simulink model "control"  (R2020a)
settings: Solver=FixedStepDiscrete  StartTime=0.0  StopTime=1  FixedStep=0.0005  RelTol=1e-3  EnableMultiTasking=on
undefined symbols (not defined in the file): acc_calmax1, acc_calmax2, acc_calmin1, acc_calmin2, akemancanshu, bre, bre_calmax, bre_calmin, ecucoder_acal, I_AN01_5K1, I_AN03_5V, I_AN04_5V, kd, ki, kp, leftmax, O_SW06_HS1A, rightmax, T_add, T_del, tiaoshi, zhiling
libraries: ec5744lib x252, canmsglib x92, simulink x5
(part 2 of 9)

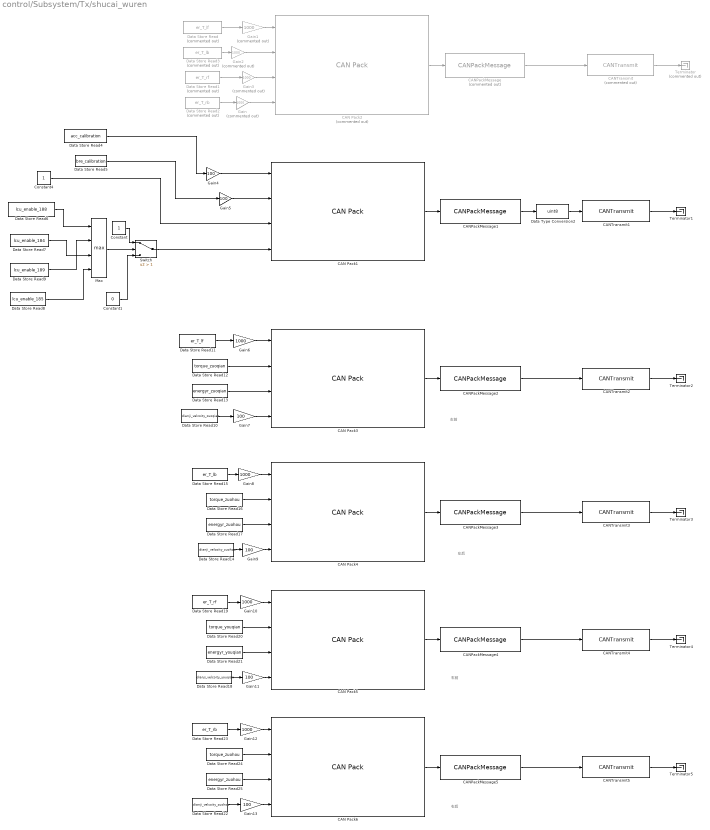
== system control/Subsystem/Tx/shucai_wuren ==
  note: 右后
  note: 右前
  note: 左后
  note: 左前
  CAN Pack1 : canmsglib/CAN Pack  CANdbFile=C:\Users\18137\Desktop\HRT\E02\HRT_23E.dbc  MsgList=(none)  MsgName=shucai  MsgIDType=Standard (11-bit identifier)  MsgIdentifier=5  MsgLength=8  Remote=off  ApplyMinMax=off  BusOutput=off  SignalInfo={'acc_signal','0','8','LE','unsigned','Standard','0','1','0','0','255';'bre_signal','8','8','LE','unsigned','Standard','0','1','0','0','255';'code_version','16','8','LE','unsigned','Standard','0','1','0','0','255';'enable_condition','24','8','LE','unsigned','Standard','0','1','0','0','255'}
      settings: SourceProductBaseCode=ME,XP,VN  DataFormat=CANdb specified signals
  CAN Pack2 : canmsglib/CAN Pack  Commented=on  CANdbFile=C:\Users\18137\Desktop\HRT\E02\HRT_23E.dbc  MsgList=(none)  MsgName=shucai_wuren  MsgIDType=Standard (11-bit identifier)  MsgIdentifier=102  MsgLength=8  Remote=off  ApplyMinMax=off  BusOutput=off  SignalInfo={'current_torque_lf','16','16','LE','signed','Standard','0','1','0','-32768','32767';'current_torque_lr','32','16','LE','signed','Standard','0','1','0','-32768','32767';'current_torque_rf','48','16','LE','signed','Standard','0','1','0','-32768','32767';'current_torque_rr','0','16','LE','signed','Standard','0','1','0','-32768','32767'}
      settings: SourceProductBaseCode=ME,XP,VN  DataFormat=CANdb specified signals
  CAN Pack{3..6} (4 alike) : canmsglib/CAN Pack  CANdbFile=C:\Users\86155\Desktop\HRT2024\qkx\can\energy_receive.dbc  MsgList=caijishuju_Copy_lf  MsgName=caijishuju_Copy_lf  MsgIDType=Standard (11-bit identifier)  MsgIdentifier=257  MsgLength=8  Remote=off  ApplyMinMax=off  BusOutput=off  SignalInfo={'current','0','16','LE','signed','Standard','0','1','0','-32768','32767';'odd_pressure','16','16','LE','signed','Standard','0','1','0','-32768','32767';'torque','32','16','LE','signed','Standard','0','1','0','-32768','32767';'velocity','48','16','LE','signed','Standard','0','1','0','-32768','32767'}
      settings: SourceProductBaseCode=ME,XP,VN  DataFormat=CANdb specified signals
  CANPackMessage : ec5744lib/RapidECU_U4B/04CANCommunication/CANPackMessage  Commented=on  datalength=8  sampletime=-1
      settings: SourceProductName=ECUCoder for MPC5744
  CANPackMessage{1..5} (5 alike) : ec5744lib/RapidECU_U4B/04CANCommunication/CANPackMessage  datalength=8  sampletime=-1
      settings: SourceProductName=ECUCoder for MPC5744
  CANTransmit : ec5744lib/RapidECU_U4B/04CANCommunication/CANTransmit  Commented=on  canmodule=1  canbuffer=8  canmessageid=hex2dec('66')  canmessagetype=Standard(11-bit ID)  datalength=8  sampletime=-1
      settings: SourceProductName=ECUCoder for MPC5744
  CANTransmit1 : ec5744lib/RapidECU_U4B/04CANCommunication/CANTransmit  canmodule=1  canbuffer=57  canmessageid=hex2dec('5')  canmessagetype=Standard(11-bit ID)  datalength=8  sampletime=-1
      settings: SourceProductName=ECUCoder for MPC5744
  CANTransmit2 : ec5744lib/RapidECU_U4B/04CANCommunication/CANTransmit  canmodule=1  canbuffer=58  canmessageid=hex2dec('100')  canmessagetype=Standard(11-bit ID)  datalength=8  sampletime=-1
      settings: SourceProductName=ECUCoder for MPC5744
  CANTransmit3 : ec5744lib/RapidECU_U4B/04CANCommunication/CANTransmit  canmodule=1  canbuffer=59  canmessageid=hex2dec('101')  canmessagetype=Standard(11-bit ID)  datalength=8  sampletime=-1
      settings: SourceProductName=ECUCoder for MPC5744
  CANTransmit4 : ec5744lib/RapidECU_U4B/04CANCommunication/CANTransmit  canmodule=1  canbuffer=60  canmessageid=hex2dec('102')  canmessagetype=Standard(11-bit ID)  datalength=8  sampletime=-1
      settings: SourceProductName=ECUCoder for MPC5744
  CANTransmit5 : ec5744lib/RapidECU_U4B/04CANCommunication/CANTransmit  canmodule=1  canbuffer=61  canmessageid=hex2dec('103')  canmessagetype=Standard(11-bit ID)  datalength=8  sampletime=-1
      settings: SourceProductName=ECUCoder for MPC5744
  Constant : Constant
  Constant1 : Constant  Value=0
  Constant4 : Constant
  Data Store Read : DataStoreRead  Commented=on  DataStoreName=er_T_lf
  Data Store Read1 : DataStoreRead  Commented=on  DataStoreName=er_T_rf
  Data Store Read10 : DataStoreRead  DataStoreName=dianji_velcoity_zuoqian
  Data Store Read11 : DataStoreRead  DataStoreName=er_T_lf
  Data Store Read12 : DataStoreRead  DataStoreName=torque_zuoqian
  Data Store Read13 : DataStoreRead  DataStoreName=energyr_zuoqian
  Data Store Read14 : DataStoreRead  DataStoreName=dianji_velcoity_zuohou
  Data Store Read15 : DataStoreRead  DataStoreName=er_T_lb
  Data Store Read16 : DataStoreRead  DataStoreName=torque_zuohou
  Data Store Read17 : DataStoreRead  DataStoreName=energyr_zuohou
  Data Store Read18 : DataStoreRead  DataStoreName=dianji_velcoity_youqian
  Data Store Read19 : DataStoreRead  DataStoreName=er_T_rf
  Data Store Read2 : DataStoreRead  Commented=on  DataStoreName=er_T_rb
  Data Store Read20 : DataStoreRead  DataStoreName=torque_youqian
  Data Store Read21 : DataStoreRead  DataStoreName=energyr_youqian
  Data Store Read22 : DataStoreRead  DataStoreName=dianji_velcoity_zuohou
  Data Store Read23 : DataStoreRead  DataStoreName=er_T_rb
  Data Store Read24 : DataStoreRead  DataStoreName=torque_zuohou
  Data Store Read25 : DataStoreRead  DataStoreName=energyr_zuohou
  Data Store Read3 : DataStoreRead  Commented=on  DataStoreName=er_T_lb
  Data Store Read4 : DataStoreRead  DataStoreName=acc_calibration
  Data Store Read5 : DataStoreRead  DataStoreName=bre_calibration
  Data Store Read6 : DataStoreRead  DataStoreName=lcu_enable_188
  Data Store Read7 : DataStoreRead  DataStoreName=lcu_enable_184
  Data Store Read8 : DataStoreRead  DataStoreName=lcu_enable_185
  Data Store Read9 : DataStoreRead  DataStoreName=lcu_enable_189
  Data Type Conversion2 : DataTypeConversion  OutDataTypeStr=uint8
  Gain{,1..3} (4 alike) : Gain  Commented=on  Gain=1000
  Gain{6,8,10,12} (4 alike) : Gain  Gain=1000
  Gain{4..5,7,9,11,13} (6 alike) : Gain  Gain=100
  Max : MinMax  Function=max  Inputs=4
  Switch : Switch  Criteria=u2 > Threshold  Threshold=1
  Terminator : Terminator  Commented=on
  Terminator{1..5} (5 alike) : Terminator
  wires:
  CANTransmit/1 -> Terminator/1
  CAN Pack2/1 -> CANPackMessage/1
  CANPackMessage/1 -> CANTransmit/1
  Data Store Read/1 -> Gain1/1
  Data Store Read3/1 -> Gain2/1
  Data Store Read1/1 -> Gain3/1
  Data Store Read2/1 -> Gain/1
  Gain/1 -> CAN Pack2/4
  Gain3/1 -> CAN Pack2/3
  Gain2/1 -> CAN Pack2/2
  Gain1/1 -> CAN Pack2/1
  Gain4/1 -> CAN Pack1/1
  Data Store Read8/1 -> Max/4
  Gain5/1 -> CAN Pack1/2
  CANPackMessage1/1 -> Data Type Conversion2/1
  Data Store Read5/1 -> Gain5/1
  Constant4/1 -> CAN Pack1/3
  Data Store Read9/1 -> Max/2
  Data Store Read6/1 -> Max/1
  Constant1/1 -> Switch/3
  CANTransmit1/1 -> Terminator1/1
  Data Store Read7/1 -> Max/3
  CAN Pack1/1 -> CANPackMessage1/1
  Max/1 -> Switch/2
  Constant/1 -> Switch/1
  Data Store Read4/1 -> Gain4/1
  Data Type Conversion2/1 -> CANTransmit1/1
  Switch/1 -> CAN Pack1/4
  CANPackMessage2/1 -> CANTransmit2/1
  CANTransmit2/1 -> Terminator2/1
  CAN Pack3/1 -> CANPackMessage2/1
  Data Store Read10/1 -> Gain7/1
  Data Store Read11/1 -> Gain6/1
  Data Store Read12/1 -> CAN Pack3/2
  Data Store Read13/1 -> CAN Pack3/3
  Data Store Read17/1 -> CAN Pack4/3
  Data Store Read14/1 -> Gain9/1
  Data Store Read15/1 -> Gain8/1
  Data Store Read16/1 -> CAN Pack4/2
  CAN Pack4/1 -> CANPackMessage3/1
  CANTransmit3/1 -> Terminator3/1
  CANPackMessage3/1 -> CANTransmit3/1
  Data Store Read21/1 -> CAN Pack5/3
  Data Store Read18/1 -> Gain11/1
  Data Store Read19/1 -> Gain10/1
  Data Store Read20/1 -> CAN Pack5/2
  CAN Pack5/1 -> CANPackMessage4/1
  CANTransmit4/1 -> Terminator4/1
  CANPackMessage4/1 -> CANTransmit4/1
  Data Store Read25/1 -> CAN Pack6/3
  Data Store Read22/1 -> Gain13/1
  Data Store Read23/1 -> Gain12/1
  Data Store Read24/1 -> CAN Pack6/2
  CAN Pack6/1 -> CANPackMessage5/1
  CANTransmit5/1 -> Terminator5/1
  CANPackMessage5/1 -> CANTransmit5/1
  Gain6/1 -> CAN Pack3/1
  Gain7/1 -> CAN Pack3/4
  Gain8/1 -> CAN Pack4/1
  Gain9/1 -> CAN Pack4/4
  Gain10/1 -> CAN Pack5/1
  Gain11/1 -> CAN Pack5/4
  Gain12/1 -> CAN Pack6/1
  Gain13/1 -> CAN Pack6/4

== system control/Subsystem/Tx/转向 ==
  Data Store Read1 : DataStoreRead  DataStoreName=match_model
  Data Store Read2 : DataStoreRead  DataStoreName=status
  Data Store Write : DataStoreWrite  DataStoreName=kp
  Data Store Write1 : DataStoreWrite  DataStoreName=ki
  Data Store Write2 : DataStoreWrite  DataStoreName=kd
  Data Store Write3 : DataStoreWrite  DataStoreName=kenable
  ECCalVar : Constant  InitFcn=ecucoder_acal;  Value=kp  OutDataTypeStr=Inherit: Inherit via back propagation  SampleTime=-1
  ECCalVar1 : Constant  InitFcn=ecucoder_acal;  Value=ki  OutDataTypeStr=Inherit: Inherit via back propagation  SampleTime=-1
  ECCalVar2 : Constant  InitFcn=ecucoder_acal;  Value=kd  OutDataTypeStr=Inherit: Inherit via back propagation  SampleTime=-1
  MATLAB Function1 : MATLAB Function  TreatAsAtomicUnit=on
  Max : MinMax  Inputs=3
  转向换算 : Subsystem
  wires:
  Data Store Read1/1 -> MATLAB Function1/1(model)
  ECCalVar1/1 -> Max/2, Data Store Write1/1
  ECCalVar2/1 -> Max/1, Data Store Write2/1
  ECCalVar/1 -> Max/3, Data Store Write/1
  Data Store Read2/1 -> MATLAB Function1/2(status)
  MATLAB Function1/1(y) -> 转向换算/Enable
  Max/1 -> Data Store Write3/1

== system control/Subsystem/run/analog_input ==
  Add : Sum
  Data Store Read{,1..3,7} (5 alike) : DataStoreRead  DataStoreName=match_model
  Data Store Read4 : DataStoreRead  DataStoreName=lcu_canok
  Data Store Read5 : DataStoreRead  DataStoreName=lcu_canok
  Data Store Read6 : DataStoreRead  DataStoreName=workstation_status
  Data Store Read8 : DataStoreRead  DataStoreName=V_workstation
  Data Store Read9 : DataStoreRead  DataStoreName=V_Kalman
  MATLAB Function : MATLAB Function  TreatAsAtomicUnit=on
  MATLAB Function1 : MATLAB Function  TreatAsAtomicUnit=on
  MATLAB Function2 : MATLAB Function  TreatAsAtomicUnit=on
  MATLAB Function3 : MATLAB Function  TreatAsAtomicUnit=on
  MATLAB Function4 : MATLAB Function  TreatAsAtomicUnit=on
  MATLAB Function5 : MATLAB Function  TreatAsAtomicUnit=on
  MATLAB Function6 : MATLAB Function  TreatAsAtomicUnit=on
  Saturation : Saturate  UpperLimit=50  LowerLimit=0
  Switch : Switch  Criteria=u2 > Threshold
  基准扭矩 : DataStoreWrite  Commented=on  DataStoreName=M
  无人意图转译 : Subsystem
  有人 : Subsystem
  bre : Outport
  acc : Outport  Port=2
  wires:
  Data Store Read1/1 -> MATLAB Function/1(u)
  MATLAB Function/1(y) -> MATLAB Function1/1(u)
  Switch/1 -> MATLAB Function1/2(a)
  有人/1(TP) -> Switch/3
  有人/2(bre) -> bre/1
  Data Store Read2/1 -> MATLAB Function2/1(u)
  MATLAB Function2/1(y) -> 有人/Enable
  Data Store Read3/1 -> MATLAB Function3/1(model)
  无人意图转译/1(Out1) -> Switch/1
  MATLAB Function3/1(y) -> 无人意图转译/Enable
  Data Store Read4/1 -> MATLAB Function3/2(canok)
  Data Store Read5/1 -> MATLAB Function2/2(canok)
  Data Store Read6/1 -> MATLAB Function4/1(u)
  MATLAB Function1/1(y) -> MATLAB Function4/2(a)
  MATLAB Function4/1(y) -> MATLAB Function5/1(u)
  Data Store Read7/1 -> MATLAB Function5/2(model)
  MATLAB Function5/2(y6) -> Saturation/1
  Saturation/1 -> Add/2
  MATLAB Function5/1(y) -> Add/1
  Add/1 -> 基准扭矩/1, acc/1
  MATLAB Function6/1(y) -> Switch/2
  Data Store Read8/1 -> MATLAB Function3/3(workstation)
  Data Store Read9/1 -> MATLAB Function3/4(v)
  Data Store Read/1 -> MATLAB Function6/1(model)

== system control/Subsystem/run/ctrl ==
  note: 控制策略所在地
  基准扭矩 : Inport
  Subsystem1 : Subsystem
  wires:
  基准扭矩/1 -> Subsystem1/1(扭矩)

== system control/无人TX1/转向自动标定/Subsystem ==
  Enable : EnablePort
  CAN Pack : canmsglib/CAN Pack  CANdbFile=C:\Users\Liu keliang\Desktop\HRT2023\HRT23赛季刘科良\CANdbc\steering.dbc  MsgList=(none)  MsgName=enable123  MsgIDType=Standard (11-bit identifier)  MsgIdentifier=291  MsgLength=1  Remote=off  ApplyMinMax=off  BusOutput=off  SignalInfo={'enable123','0','8','LE','unsigned','Standard','0','1','0','0','255'}
      settings: SourceProductBaseCode=ME,XP,VN  DataFormat=CANdb specified signals
  CAN Pack1 : canmsglib/CAN Pack  CANdbFile=C:\Users\Liu keliang\Desktop\HRT2023\HRT23赛季刘科良\CANdbc\steering.dbc  MsgList=(none)  MsgName=enable0  MsgIDType=Standard (11-bit identifier)  MsgIdentifier=0  MsgLength=8  Remote=off  ApplyMinMax=off  BusOutput=off  SignalInfo={'enable_00','0','16','LE','unsigned','Standard','0','1','0','0','65535';'enable_00_Copy_1','16','16','LE','unsigned','Standard','0','1','0','0','65535';'enable_00_Copy_2','32','16','LE','unsigned','Standard','0','1','0','0','65535';'enable_00_Copy_3','48','16','LE','unsigned','Standard','0','1','0','0','65535'}
      settings: SourceProductBaseCode=ME,XP,VN  DataFormat=CANdb specified signals
  CAN Pack2 : canmsglib/CAN Pack  CANdbFile=C:\Users\Liu keliang\Desktop\HRT2023\HRT23赛季刘科良\CANdbc\steering.dbc  MsgList=(none)  MsgName=enable401  MsgIDType=Standard (11-bit identifier)  MsgIdentifier=1025  MsgLength=6  Remote=off  ApplyMinMax=off  BusOutput=off  SignalInfo={'enable401','0','8','LE','unsigned','Standard','0','1','0','0','255';'enable401_Copy_1','8','8','LE','unsigned','Standard','0','1','0','0','255';'enable401_Copy_2','16','32','LE','signed','Standard','0','1','0','-2147483648','2147483647'}
      settings: SourceProductBaseCode=ME,XP,VN  DataFormat=CANdb specified signals
  CAN Pack4 : canmsglib/CAN Pack  CANdbFile=C:\Users\Liu keliang\Desktop\HRT2023\HRT23赛季刘科良\CANdbc\steering.dbc  MsgList=(none)  MsgName=enable80  MsgIDType=Standard (11-bit identifier)  MsgIdentifier=128  MsgLength=1  Remote=off  ApplyMinMax=off  BusOutput=off  SignalInfo={'dingshi','0','8','LE','unsigned','Standard','0','1','0','0','255'}
      settings: SourceProductBaseCode=ME,XP,VN  DataFormat=CANdb specified signals
  CANPackMessage : ec5744lib/RapidECU_U4B/04CANCommunication/CANPackMessage  datalength=1  sampletime=-1
      settings: SourceProductName=ECUCoder for MPC5744
  CANPackMessage1 : ec5744lib/RapidECU_U4B/04CANCommunication/CANPackMessage  datalength=8  sampletime=-1
      settings: SourceProductName=ECUCoder for MPC5744
  CANPackMessage2 : ec5744lib/RapidECU_U4B/04CANCommunication/CANPackMessage  datalength=6  sampletime=-1
      settings: SourceProductName=ECUCoder for MPC5744
  CANPackMessage4 : ec5744lib/RapidECU_U4B/04CANCommunication/CANPackMessage  datalength=1  sampletime=-1
      settings: SourceProductName=ECUCoder for MPC5744
  CANTransmit : ec5744lib/RapidECU_U4B/04CANCommunication/CANTransmit  canmodule=2  canbuffer=15  canmessageid=hex2dec('123')  canmessagetype=Standard(11-bit ID)  datalength=1  sampletime=-1
      settings: SourceProductName=ECUCoder for MPC5744
  CANTransmit1 : ec5744lib/RapidECU_U4B/04CANCommunication/CANTransmit  canmodule=2  canbuffer=56  canmessageid=hex2dec('00')  canmessagetype=Standard(11-bit ID)  datalength=8  sampletime=-1
      settings: SourceProductName=ECUCoder for MPC5744
  CANTransmit2 : ec5744lib/RapidECU_U4B/04CANCommunication/CANTransmit  canmodule=2  canbuffer=57  canmessageid=hex2dec('401')  canmessagetype=Standard(11-bit ID)  datalength=6  sampletime=-1
      settings: SourceProductName=ECUCoder for MPC5744
  CANTransmit4 : ec5744lib/RapidECU_U4B/04CANCommunication/CANTransmit  canmodule=2  canbuffer=58  canmessageid=hex2dec('80')  canmessagetype=Standard(11-bit ID)  datalength=1  sampletime=-1
      settings: SourceProductName=ECUCoder for MPC5744
  Constant : Constant  Value=0  SampleTime=-1
  Constant1 : Constant  SampleTime=-1
  Constant{2..4,6} (4 alike) : Constant  Value=0
  Constant5 : Constant  Value=0  SampleTime=-1
  Data Store Read : DataStoreRead  DataStoreName=zhuanjiaobianmaqi
  Data Store Read1 : DataStoreRead  DataStoreName=rm
  Data Store Read2 : DataStoreRead  DataStoreName=lm
  Data Type Conversion : DataTypeConversion  OutDataTypeStr=uint8
  Data Type Conversion1 : DataTypeConversion  OutDataTypeStr=uint8
  Data Type Conversion2 : DataTypeConversion  Commented=on  OutDataTypeStr=uint8
  Data Type Conversion3 : DataTypeConversion  OutDataTypeStr=single
  Data Type Conversion4 : DataTypeConversion  OutDataTypeStr=uint8
  Data Type Conversion5 : DataTypeConversion  OutDataTypeStr=single
  Data Type Conversion6 : DataTypeConversion  OutDataTypeStr=single
  FRAMEnable : ec5744lib/RapidECU_U4B/12EEModule/FRAMEnable  framenable=on
      settings: SourceProductName=ECUCoder for MPC5744
  FRAMWrite : ec5744lib/RapidECU_U4B/12EEModule/FRAMWrite  buffer=0  sampletime=-1
      settings: SourceProductName=ECUCoder for MPC5744
  FRAMWrite1 : ec5744lib/RapidECU_U4B/12EEModule/FRAMWrite  buffer=1  sampletime=-1
      settings: SourceProductName=ECUCoder for MPC5744
  FRAMWrite2 : ec5744lib/RapidECU_U4B/12EEModule/FRAMWrite  buffer=10  sampletime=-1
      settings: SourceProductName=ECUCoder for MPC5744
  FRAMWrite3 : ec5744lib/RapidECU_U4B/12EEModule/FRAMWrite  buffer=11  sampletime=-1
      settings: SourceProductName=ECUCoder for MPC5744
  MATLAB Function : MATLAB Function  TreatAsAtomicUnit=on
  MeaModule : ec5744lib/RapidECU_U4B/07Calibration/MeaModule  signal=msk
      settings: SourceProductName=ECUCoder for MPC5744
  MeaModule1 : ec5744lib/RapidECU_U4B/07Calibration/MeaModule  signal=msd
      settings: SourceProductName=ECUCoder for MPC5744
  Terminator{,1..2,4} (4 alike) : Terminator
  Zero-Order Hold{,1..4} (5 alike) : ZeroOrderHold  SampleTime=-1
  wires:
  CANTransmit/1 -> Terminator/1
  Zero-Order Hold2/1 -> CAN Pack1/3
  MATLAB Function/2(y) -> CAN Pack2/1
  CAN Pack1/1 -> CANPackMessage1/1
  CANTransmit2/1 -> Terminator2/1
  CANPackMessage4/1 -> Data Type Conversion4/1
  CAN Pack2/1 -> CANPackMessage2/1
  CANTransmit1/1 -> Terminator1/1
  Constant/1 -> Zero-Order Hold/1
  Data Type Conversion1/1 -> CANTransmit1/1
  Constant6/1 -> CAN Pack2/2
  CANTransmit4/1 -> Terminator4/1
  Data Type Conversion/1 -> CANTransmit/1
  Zero-Order Hold/1 -> CAN Pack/1
  CANPackMessage/1 -> Data Type Conversion/1
  Data Type Conversion4/1 -> CANTransmit4/1
  Constant4/1 -> Zero-Order Hold3/1
  CAN Pack/1 -> CANPackMessage/1
  CANPackMessage1/1 -> Data Type Conversion1/1
  Constant5/1 -> Zero-Order Hold4/1
  CAN Pack4/1 -> CANPackMessage4/1
  Constant3/1 -> Zero-Order Hold2/1
  Constant2/1 -> Zero-Order Hold1/1
  Constant1/1 -> CAN Pack1/1
  Zero-Order Hold4/1 -> CAN Pack4/1
  Zero-Order Hold1/1 -> CAN Pack1/2
  CANPackMessage2/1 -> CANTransmit2/1
  Zero-Order Hold3/1 -> CAN Pack1/4
  MATLAB Function/1(steer) -> CAN Pack2/3
  Data Store Read/1 -> Data Type Conversion3/1
  MATLAB Function/3(k) -> MeaModule/1
  Data Store Read1/1 -> FRAMWrite2/1, MATLAB Function/1(rm)
  Data Store Read2/1 -> FRAMWrite3/1, MATLAB Function/2(lm)
  Data Type Conversion3/1 -> MATLAB Function/3(bianmaqi)
  MATLAB Function/4(d) -> MeaModule1/1
  MeaModule1/1 -> Data Type Conversion5/1
  Data Type Conversion5/1 -> FRAMWrite1/1
  Data Type Conversion6/1 -> FRAMWrite/1
  MeaModule/1 -> Data Type Conversion6/1

== system control/无人TX1/转向自动标定/Subsystem1 ==
  y1 : Inport
  y2 : Inport  Port=2
  Enable : EnablePort
  CAN Pack5 : canmsglib/CAN Pack  CANdbFile=C:\Users\Liu keliang\Desktop\HRT2023\HRT23赛季刘科良\CANdbc\zhuanxiangresetting.dbc  MsgList=(none)  MsgName=reseting  MsgIDType=Standard (11-bit identifier)  MsgIdentifier=1537  MsgLength=8  Remote=off  ApplyMinMax=off  BusOutput=off  SignalInfo={'reseting1','0','32','LE','unsigned','Standard','0','1','0','-Inf','Inf';'reseting2','32','32','LE','unsigned','Standard','0','1','0','-Inf','Inf'}
      settings: SourceProductBaseCode=ME,XP,VN  DataFormat=CANdb specified signals
  CANPackMessage3 : ec5744lib/RapidECU_U4B/04CANCommunication/CANPackMessage  datalength=8  sampletime=-1
      settings: SourceProductName=ECUCoder for MPC5744
  CANTransmit3 : ec5744lib/RapidECU_U4B/04CANCommunication/CANTransmit  canmodule=2  canbuffer=60  canmessageid=hex2dec('601')  canmessagetype=Standard(11-bit ID)  datalength=8  sampletime=-1
      settings: SourceProductName=ECUCoder for MPC5744
  Data Type Conversion3 : DataTypeConversion  OutDataTypeStr=uint8
  Terminator3 : Terminator
  wires:
  CAN Pack5/1 -> CANPackMessage3/1
  y1/1 -> CAN Pack5/1
  CANTransmit3/1 -> Terminator3/1
  Data Type Conversion3/1 -> CANTransmit3/1
  CANPackMessage3/1 -> Data Type Conversion3/1
  y2/1 -> CAN Pack5/2

== system control/Subsystem/Rx/283 285左前/Subsystem1 ==
  Enable : Inport
  ID : Inport  Port=2
  msg : Inport  Port=3
  function : TriggerPort  TriggerType=function-call  VariantControl=Variant
  Subsystem : Subsystem
  wires:
  ID/1 -> Subsystem/1(ID)
  msg/1 -> Subsystem/2(msg)
  Enable/1 -> Subsystem/Enable

== system control/Subsystem/Rx/283 285左前/Subsystem2 ==
  Enable : Inport
  ID : Inport  Port=2
  msg : Inport  Port=3
  function : TriggerPort  TriggerType=function-call  VariantControl=Variant
  Subsystem : Subsystem
  wires:
  ID/1 -> Subsystem/1(ID)
  msg/1 -> Subsystem/2(msg)
  Enable/1 -> Subsystem/Enable

== system control/Subsystem/Rx/284 286右前/Subsystem1 ==
  Enable : Inport
  ID : Inport  Port=2
  msg : Inport  Port=3
  function : TriggerPort  TriggerType=function-call  VariantControl=Variant
  Subsystem : Subsystem
  wires:
  ID/1 -> Subsystem/1(ID)
  msg/1 -> Subsystem/2(msg)
  Enable/1 -> Subsystem/Enable

== system control/Subsystem/Rx/284 286右前/Subsystem2 ==
  Enable : Inport
  ID : Inport  Port=2
  msg : Inport  Port=3
  function : TriggerPort  TriggerType=function-call  VariantControl=Variant
  Subsystem : Subsystem
  wires:
  ID/1 -> Subsystem/1(ID)
  msg/1 -> Subsystem/2(msg)
  Enable/1 -> Subsystem/Enable

== system control/Subsystem/Rx/287 289右后/Subsystem1 ==
  Enable : Inport
  ID : Inport  Port=2
  msg : Inport  Port=3
  function : TriggerPort  TriggerType=function-call  VariantControl=Variant
  Subsystem : Subsystem
  wires:
  ID/1 -> Subsystem/1(ID)
  msg/1 -> Subsystem/2(msg)
  Enable/1 -> Subsystem/Enable

== system control/Subsystem/Rx/287 289右后/Subsystem3 ==
  Enable : Inport
  ID : Inport  Port=2
  msg : Inport  Port=3
  function : TriggerPort  TriggerType=function-call  VariantControl=Variant
  Subsystem : Subsystem
  wires:
  ID/1 -> Subsystem/1(ID)
  msg/1 -> Subsystem/2(msg)
  Enable/1 -> Subsystem/Enable

== system control/Subsystem/Rx/288 290左后/Subsystem1 ==
  Enable : Inport
  ID : Inport  Port=2
  msg : Inport  Port=3
  function : TriggerPort  TriggerType=function-call  VariantControl=Variant
  Subsystem : Subsystem
  wires:
  ID/1 -> Subsystem/1(ID)
  msg/1 -> Subsystem/2(msg)
  Enable/1 -> Subsystem/Enable

== system control/Subsystem/Rx/288 290左后/Subsystem2 ==
  Enable : Inport
  ID : Inport  Port=2
  msg : Inport  Port=3
  function : TriggerPort  TriggerType=function-call  VariantControl=Variant
  Subsystem : Subsystem
  wires:
  ID/1 -> Subsystem/1(ID)
  msg/1 -> Subsystem/2(msg)
  Enable/1 -> Subsystem/Enable

== system control/Subsystem/Rx/ebs/Subsystem3 ==
  Enable : Inport
  ID : Inport  Port=2
  msg : Inport  Port=3
  function : TriggerPort  TriggerType=function-call  VariantControl=Variant
  Subsystem : Subsystem
  wires:
  ID/1 -> Subsystem/1(ID)
  msg/1 -> Subsystem/2(msg)
  Enable/1 -> Subsystem/Enable

== system control/Subsystem/Rx/lcu——receive/Subsystem1 ==
  Enable : Inport
  ID : Inport  Port=2
  msg : Inport  Port=3
  function : TriggerPort  TriggerType=function-call  VariantControl=Variant
  Subsystem : Subsystem
  m : Outport
  wires:
  ID/1 -> Subsystem/1(ID)
  msg/1 -> Subsystem/2(msg)
  Enable/1 -> Subsystem/Enable
  Subsystem/1(CAN_msg_enable) -> m/1

== system control/Subsystem/Rx/工作站/Subsystem1 ==
  Enable : Inport
  ID : Inport  Port=2
  msg : Inport  Port=3
  function : TriggerPort  TriggerType=function-call  VariantControl=Variant
  Subsystem1 : Subsystem
  wires:
  Enable/1 -> Subsystem1/Enable
  ID/1 -> Subsystem1/1(ID)
  msg/1 -> Subsystem1/2(msg)

== system control/Subsystem/Rx/工作站/Subsystem3 ==
  Enable : Inport
  ID : Inport  Port=2
  msg : Inport  Port=3
  function : TriggerPort  TriggerType=function-call  VariantControl=Variant
  Subsystem : Subsystem
  wires:
  ID/1 -> Subsystem/1(ID)
  msg/1 -> Subsystem/2(msg)
  Enable/1 -> Subsystem/Enable

== system control/Subsystem/Rx/惯导/Subsystem1 ==
  Enable : Inport
  ID : Inport  Port=2
  msg : Inport  Port=3
  function : TriggerPort  TriggerType=function-call  VariantControl=Variant
  Subsystem : Subsystem
  wires:
  ID/1 -> Subsystem/1(ID)
  msg/1 -> Subsystem/2(msg)
  Enable/1 -> Subsystem/Enable

== system control/Subsystem/Rx/惯导/Subsystem2 ==
  Enable : Inport
  ID : Inport  Port=2
  msg : Inport  Port=3
  function : TriggerPort  TriggerType=function-call  VariantControl=Variant
  Subsystem : Subsystem
  wires:
  ID/1 -> Subsystem/1(ID)
  msg/1 -> Subsystem/2(msg)
  Enable/1 -> Subsystem/Enable

== system control/Subsystem/Rx/惯导/Subsystem3 ==
  Enable : Inport
  ID : Inport  Port=2
  msg : Inport  Port=3
  function : TriggerPort  TriggerType=function-call  VariantControl=Variant
  Subsystem : Subsystem
  wires:
  ID/1 -> Subsystem/1(ID)
  msg/1 -> Subsystem/2(msg)
  Enable/1 -> Subsystem/Enable

== system control/Subsystem/Rx/转向——receive1/Subsystem1 ==
  Enable : Inport
  ID : Inport  Port=2
  msg : Inport  Port=3
  function : TriggerPort  TriggerType=function-call  VariantControl=Variant
  Subsystem : Subsystem
  wires:
  ID/1 -> Subsystem/1(ID)
  msg/1 -> Subsystem/2(msg)
  Enable/1 -> Subsystem/Enable

== system control/Subsystem/Rx/转向——receive1/Subsystem3 ==
  Enable : Inport
  ID : Inport  Port=2
  msg : Inport  Port=3
  function : TriggerPort  TriggerType=function-call  VariantControl=Variant
  Subsystem : Subsystem
  wires:
  ID/1 -> Subsystem/1(ID)
  msg/1 -> Subsystem/2(msg)
  Enable/1 -> Subsystem/Enable

== system control/Subsystem/Rx/转向——receive编码器/Subsystem3 ==
  Enable : Inport
  ID : Inport  Port=2
  msg : Inport  Port=3
  function : TriggerPort  TriggerType=function-call  VariantControl=Variant
  Subsystem : Subsystem
  wires:
  ID/1 -> Subsystem/1(ID)
  msg/1 -> Subsystem/2(msg)
  Enable/1 -> Subsystem/Enable

== system control/Subsystem/Tx/TX控制器/Subsystem1 ==
  angle : Inport
  v : Inport  Port=2
  Data Store Read4 : DataStoreRead  DataStoreName=match_model
  ECCalVar : Constant  InitFcn=ecucoder_acal;  Value=akemancanshu  OutDataTypeStr=Inherit: Inherit via back propagation  SampleTime=-1
  MATLAB Function2 : MATLAB Function  TreatAsAtomicUnit=on
  youqianvvv : Outport
  zuoqianvvv : Outport  Port=2
  youhouvvv : Outport  Port=3
  zuohouvvv : Outport  Port=4
  wires:
  MATLAB Function2/2(zuoqianvvv) -> zuoqianvvv/1
  v/1 -> MATLAB Function2/2(v)
  MATLAB Function2/1(youqianvvv) -> youqianvvv/1
  MATLAB Function2/3(youhouvvv) -> youhouvvv/1
  angle/1 -> MATLAB Function2/1(anglenb)
  MATLAB Function2/4(zuohouvvv) -> zuohouvvv/1
  Data Store Read4/1 -> MATLAB Function2/3(model)
  ECCalVar/1 -> MATLAB Function2/4(k)

== system control/Subsystem/Tx/TX控制器/扭矩 ==
  note: 185右前 284 286
  note: 188右后 287 289
  note: 184左前 283 285
  note: 189左后 288 290
  Enable : EnablePort
  184左前 : Subsystem
  185右前 : Subsystem
  188右后 : Subsystem
  189左后 : Subsystem
  TEST : Subsystem  Commented=on

== system control/Subsystem/Tx/TX控制器/速度 ==
  note: 185右前 284 286
  note: 188右后 287 289
  note: 184左前 283 285
  note: 189左后 288 290
  Enable : EnablePort
  184左前 : Subsystem
  185右前 : Subsystem
  188右后 : Subsystem
  189左后 : Subsystem

== system control/Subsystem/Tx/TX控制器/速度1 ==
  note: 189左后 288 290
  note: 184左前 283 285
  note: 188右后 287 289
  note: 185右前 284 286
  Enable : EnablePort
  184左前 : Subsystem
  185右前 : Subsystem
  188右后 : Subsystem
  189左后 : Subsystem

== system control/Subsystem/Tx/Toworkstation/toworkstation ==
  Enable : EnablePort
  toworkstation : Subsystem

== system control/Subsystem/Tx/Toworkstation/转向 ==
  Data Store Read : DataStoreRead  DataStoreName=match_model
  MATLAB Function : MATLAB Function  TreatAsAtomicUnit=on
  Subsystem : Subsystem
  wires:
  Data Store Read/1 -> MATLAB Function/1(u)
  MATLAB Function/1(y) -> Subsystem/Enable

== system control/Subsystem/Tx/esc，ABS/Subsystem ==
  Enable : EnablePort
  CAN Pack : canmsglib/CAN Pack  CANdbFile=C:\Users\Liu keliang\Desktop\HRT2023\HRT23赛季刘科良\CANdbc\esc.dbc  MsgList=(none)  MsgName=esc  MsgIDType=Standard (11-bit identifier)  MsgIdentifier=1638  MsgLength=8  Remote=off  ApplyMinMax=off  BusOutput=off  SignalInfo={'youhou','0','16','LE','unsigned','Standard','0','1','0','0','65535';'youqian','16','16','LE','unsigned','Standard','0','1','0','0','65535';'zuohou','32','16','LE','unsigned','Standard','0','1','0','0','65535';'zuoqian','48','16','LE','unsigned','Standard','0','1','0','0','65535'}
      settings: SourceProductBaseCode=ME,XP,VN  DataFormat=CANdb specified signals
  CANPackMessage : ec5744lib/RapidECU_U4B/04CANCommunication/CANPackMessage  datalength=8  sampletime=-1
      settings: SourceProductName=ECUCoder for MPC5744
  CANTransmit : ec5744lib/RapidECU_U4B/04CANCommunication/CANTransmit  canmodule=2  canbuffer=12  canmessageid=hex2dec('666')  canmessagetype=Standard(11-bit ID)  datalength=8  sampletime=-1
      settings: SourceProductName=ECUCoder for MPC5744
  Data Store Read : DataStoreRead  DataStoreName=oral_pressure_leftbehind
  Data Store Read1 : DataStoreRead  DataStoreName=oral_pressure_rightbehind
  Data Store Read2 : DataStoreRead  DataStoreName=oral_pressure_rightfront
  Data Store Read3 : DataStoreRead  DataStoreName=oral_pressure_leftfront
  Data Store Read4 : DataStoreRead  DataStoreName=brake_slipzuohou
  Data Store Read5 : DataStoreRead  DataStoreName=brake_slipyouhou
  Data Store Read6 : DataStoreRead  DataStoreName=brake_slipyouqian
  Data Store Read7 : DataStoreRead  DataStoreName=brake_slipzuoqian
  Data Store Read8 : DataStoreRead  DataStoreName=workstation_status
  Data Type Conversion : DataTypeConversion  OutDataTypeStr=uint8
  MATLAB Function : MATLAB Function  TreatAsAtomicUnit=on
  MATLAB Function1 : MATLAB Function  TreatAsAtomicUnit=on
  MATLAB Function2 : MATLAB Function  TreatAsAtomicUnit=on
  MATLAB Function3 : MATLAB Function  TreatAsAtomicUnit=on
  Max{,1..3} (4 alike) : MinMax  Function=max  Inputs=2
  MeaModule : ec5744lib/RapidECU_U4B/07Calibration/MeaModule  signal=esc
      settings: SourceProductName=ECUCoder for MPC5744
  Terminator : Terminator
  wires:
  CAN Pack/1 -> CANPackMessage/1
  CANTransmit/1 -> MeaModule/1
  Data Type Conversion/1 -> CANTransmit/1
  CANPackMessage/1 -> Data Type Conversion/1
  MeaModule/1 -> Terminator/1
  Data Store Read5/1 -> Max/1
  Data Store Read1/1 -> Max/2
  Data Store Read2/1 -> Max1/1
  Data Store Read6/1 -> Max1/2
  Data Store Read/1 -> Max2/1
  Data Store Read4/1 -> Max2/2
  Data Store Read7/1 -> Max3/1
  Data Store Read3/1 -> Max3/2
  Data Store Read8/1 -> MATLAB Function/2(status), MATLAB Function1/2(status), MATLAB Function2/2(status), MATLAB Function3/2(status)
  Max1/1 -> MATLAB Function1/1(u)
  Max2/1 -> MATLAB Function2/1(u)
  Max3/1 -> MATLAB Function3/1(u)
  MATLAB Function/1(y) -> CAN Pack/1
  MATLAB Function1/1(y) -> CAN Pack/2
  MATLAB Function2/1(y) -> CAN Pack/3
  MATLAB Function3/1(y) -> CAN Pack/4
  Max/1 -> MATLAB Function/1(u)

== system control/Subsystem/Tx/转向/转向换算 ==
  Enable : EnablePort
  Data Store Read : DataStoreRead  DataStoreName=zhuanxiangbaocuo
  Data Store Read1 : DataStoreRead  DataStoreName=zhuanxiangbaocuo
  MATLAB Function : MATLAB Function  TreatAsAtomicUnit=on
  MATLAB Function1 : MATLAB Function  TreatAsAtomicUnit=on
  Subsystem : Subsystem
  Subsystem1 : Subsystem
  wires:
  MATLAB Function/1(biaozhi1) -> Subsystem/Enable
  MATLAB Function1/3(biaozhi2) -> Subsystem1/Enable
  MATLAB Function1/2(y2) -> Subsystem1/2(y2)
  MATLAB Function1/1(y1) -> Subsystem1/1(y1)
  Data Store Read/1 -> MATLAB Function1/1(baocuo)
  Data Store Read1/1 -> MATLAB Function/1(baocuo)

== system control/Subsystem/run/analog_input/无人意图转译 ==
  note: 输出基准转矩
  Enable : EnablePort
  Data Store Read : DataStoreRead  DataStoreName=CANOK_20
  Saturation : Saturate  UpperLimit=1300  LowerLimit=0
  无人 : Subsystem
  计算期望扭矩 : MATLAB Function  TreatAsAtomicUnit=on
  Out1 : Outport
  wires:
  无人/1(期望纵向加速度) -> 计算期望扭矩/1(u)
  计算期望扭矩/1(y) -> Saturation/1
  Saturation/1 -> Out1/1
  Data Store Read/1 -> 计算期望扭矩/2(canok)

== system control/Subsystem/run/analog_input/有人 ==
  note: 加速踏板信号转化为0-1范围
      | 即开度
  Enable : EnablePort
  Data Store Write : DataStoreWrite  DataStoreName=yourenniuju
  MeaModule9 : ec5744lib/RapidECU_U4B/07Calibration/MeaModule  signal=tttttttt
      settings: SourceProductName=ECUCoder for MPC5744
  Subsystem : Subsystem
  Subsystem1 : Subsystem
  TP : Outport
  bre : Outport  Port=2
  wires:
  Subsystem/2(bre) -> bre/1
  Subsystem/1(acc) -> Subsystem1/1(acc_signal)
  Subsystem1/1(TP) -> MeaModule9/1
  MeaModule9/1 -> Data Store Write/1, TP/1

== system control/Subsystem/run/ctrl/Subsystem1 ==
  扭矩 : Inport
  Data Store Write : DataStoreWrite  DataStoreName=Tzuoqian
  Data Store Write1 : DataStoreWrite  DataStoreName=Tyouhou
  Data Store Write2 : DataStoreWrite  DataStoreName=Tzuohou
  Data Store Write3 : DataStoreWrite  DataStoreName=Tyouqian
  control_strategy : Subsystem
  wires:
  control_strategy/3(zuohou) -> Data Store Write2/1
  扭矩/1 -> control_strategy/1(TP)
  control_strategy/2(youqian) -> Data Store Write3/1
  control_strategy/1(youhou) -> Data Store Write1/1
  control_strategy/4(zuoqian) -> Data Store Write/1

== system control/Subsystem/Rx/283 285左前/Subsystem1/Subsystem ==
  ID : Inport
  msg : Inport  Port=2
  Enable : EnablePort
  CAN Pack : canmsglib/CAN Pack  Commented=on  CANdbFile=D:\desktop\enable.dbc  MsgList=(none)  MsgName=AMK_ActualValue1  MsgIDType=Standard (11-bit identifier)  MsgIdentifier=643  MsgLength=8  Remote=off  ApplyMinMax=off  BusOutput=off  SignalInfo={'AMK_ActualVelocity','16','16','LE','signed','Standard','0','1','0','0','65535';'AMK_MagnetizingCurrent','48','16','LE','signed','Standard','0','1','0','0','65535';'AMK_TorqueCurrent','32','16','LE','signed','Standard','0','1','0','0','65535';'AMK_bDcOn1','12','1','LE','unsigned','Standard','0','1','0','0','1';'AMK_bDerating1','15','1','LE','unsigned','Standard','0','1','0','0','1';'AMK_bError1','9','1','LE','unsigned','Standard','0','1','0','0','1';'AMK_bInverterOn1','14','1','LE','unsigned','Standard','0','1','0','0','1';'AMK_bQuitDcOn1','11','1','LE','unsigned','Standard','0','1','0','0','1';'AMK_bQuitInverterOn1','13','1','LE','unsigned','Standard','0','1','0','0','1';'AMK_bReserve1','0','8','LE','unsigned','Standard','0','1','0','0','255';'AMK_bSystemReady1','8','1','LE','unsigned','Standard','0','1','0','0','1';'AMK_bWarn1','10','1','LE','unsigned','Standard','0','1','0','0','1'}
      settings: SourceProductBaseCode=ME,XP,VN  DataFormat=CANdb specified signals
  CAN Unpack : canmsglib/CAN Unpack  CANdbFile=C:\Users\86155\Desktop\HRT2024\qkx\can\enable.dbc  MsgList=AMK_ActualValue2  MsgName=AMK_ActualValue2  MsgIDType=Standard (11-bit identifier)  MsgIdentifier=645  MsgLength=8  SignalInfo={'AMK_ErrorInfo','32','16','LE','unsigned','Standard','0','1','0','0','65535';'AMK_TempIGBT','48','16','LE','signed','Standard','0','1','0','-32768','32767';'AMK_TempInverter','16','16','LE','signed','Standard','0','1','0','-32768','32767';'AMK_TempMotor','0','16','LE','signed','Standard','0','1','0','-32768','32767'}  IDPort=off  TimestampPort=off  ErrorPort=off  RemotePort=off  LengthPort=off  StatusPort=off  ApplyMinMax=off
      settings: SourceProductBaseCode=ME,XP,VN  DataFormat=CANdb specified signals
  CANPackMessage : ec5744lib/RapidECU_U4B/04CANCommunication/CANPackMessage  Commented=on  datalength=8  sampletime=-1
      settings: SourceProductName=ECUCoder for MPC5744
  CANUnPackMessage : ec5744lib/RapidECU_U4B/04CANCommunication/CANUnPackMessage  datalength=8  canmessagetype=Standard(11-bit ID)  sampletime=-1
      settings: SourceProductName=ECUCoder for MPC5744
  wires:
  msg/1 -> CANUnPackMessage/2
  CANUnPackMessage/1 -> CAN Unpack/1
  ID/1 -> CANUnPackMessage/1
  CANPackMessage/1 -> ?
  CAN Pack/1 -> CANPackMessage/1

== system control/Subsystem/Rx/283 285左前/Subsystem2/Subsystem ==
  ID : Inport
  msg : Inport  Port=2
  Enable : EnablePort
  CAN Pack : canmsglib/CAN Pack  Commented=on  CANdbFile=D:\desktop\enable.dbc  MsgList=(none)  MsgName=AMK_ActualValue1  MsgIDType=Standard (11-bit identifier)  MsgIdentifier=643  MsgLength=8  Remote=off  ApplyMinMax=off  BusOutput=off  SignalInfo={'AMK_ActualVelocity','16','16','LE','signed','Standard','0','1','0','0','65535';'AMK_MagnetizingCurrent','48','16','LE','signed','Standard','0','1','0','0','65535';'AMK_TorqueCurrent','32','16','LE','signed','Standard','0','1','0','0','65535';'AMK_bDcOn1','12','1','LE','unsigned','Standard','0','1','0','0','1';'AMK_bDerating1','15','1','LE','unsigned','Standard','0','1','0','0','1';'AMK_bError1','9','1','LE','unsigned','Standard','0','1','0','0','1';'AMK_bInverterOn1','14','1','LE','unsigned','Standard','0','1','0','0','1';'AMK_bQuitDcOn1','11','1','LE','unsigned','Standard','0','1','0','0','1';'AMK_bQuitInverterOn1','13','1','LE','unsigned','Standard','0','1','0','0','1';'AMK_bReserve1','0','8','LE','unsigned','Standard','0','1','0','0','255';'AMK_bSystemReady1','8','1','LE','unsigned','Standard','0','1','0','0','1';'AMK_bWarn1','10','1','LE','unsigned','Standard','0','1','0','0','1'}
      settings: SourceProductBaseCode=ME,XP,VN  DataFormat=CANdb specified signals
  CAN Unpack : canmsglib/CAN Unpack  CANdbFile=C:\Users\86155\Desktop\HRT2024\qkx\can\enable.dbc  MsgList=AMK_ActualValue1  MsgName=AMK_ActualValue1  MsgIDType=Standard (11-bit identifier)  MsgIdentifier=643  MsgLength=8  SignalInfo={'AMK_ActualVelocity','16','16','LE','signed','Standard','0','1','0','-32768','32767';'AMK_MagnetizingCurrent','48','16','LE','signed','Standard','0','1','0','-32768','32767';'AMK_TorqueCurrent','32','16','LE','signed','Standard','0','1','0','-32768','32767';'AMK_bDcOn1','12','1','LE','unsigned','Standard','0','1','0','0','1';'AMK_bDerating1','15','1','LE','unsigned','Standard','0','1','0','0','1';'AMK_bError1','9','1','LE','unsigned','Standard','0','1','0','0','1';'AMK_bInverterOn1','14','1','LE','unsigned','Standard','0','1','0','0','1';'AMK_bQuitDcOn1','11','1','LE','unsigned','Standard','0','1','0','0','1';'AMK_bQuitInverterOn1','13','1','LE','unsigned','Standard','0','1','0','0','1';'AMK_bReserve1','0','8','LE','unsigned','Standard','0','1','0','0','255';'AMK_bSystemReady1','8','1','LE','unsigned','Standard','0','1','0','0','1';'AMK_bWarn1','10','1','LE','unsigned','Standard','0','1','0','0','1'}  IDPort=off  TimestampPort=off  ErrorPort=off  RemotePort=off  LengthPort=off  StatusPort=off  ApplyMinMax=off
      settings: SourceProductBaseCode=ME,XP,VN  DataFormat=CANdb specified signals
  CANPackMessage : ec5744lib/RapidECU_U4B/04CANCommunication/CANPackMessage  Commented=on  datalength=8  sampletime=-1
      settings: SourceProductName=ECUCoder for MPC5744
  CANUnPackMessage : ec5744lib/RapidECU_U4B/04CANCommunication/CANUnPackMessage  datalength=8  canmessagetype=Standard(11-bit ID)  sampletime=-1
      settings: SourceProductName=ECUCoder for MPC5744
  Data Store Write : DataStoreWrite  DataStoreName=dianji_velcoity_zuoqian
  Data Store Write1 : DataStoreWrite  DataStoreName=er_v_lf
  Data Store Write2 : DataStoreWrite  DataStoreName=er_T_lf
  MATLAB Function : MATLAB Function  TreatAsAtomicUnit=on
  wires:
  msg/1 -> CANUnPackMessage/2
  CANUnPackMessage/1 -> CAN Unpack/1
  ID/1 -> CANUnPackMessage/1
  CANPackMessage/1 -> ?
  CAN Unpack/1 -> MATLAB Function/1(u), Data Store Write1/1
  MATLAB Function/1(y) -> Data Store Write/1
  CAN Unpack/2 -> CAN Pack/2
  CAN Unpack/4 -> CAN Pack/5
  CAN Unpack/6 -> CAN Pack/8
  CAN Unpack/8 -> CAN Pack/11
  CAN Unpack/3 -> Data Store Write2/1

== system control/Subsystem/Rx/284 286右前/Subsystem1/Subsystem ==
  ID : Inport
  msg : Inport  Port=2
  Enable : EnablePort
  CAN Pack : canmsglib/CAN Pack  Commented=on  CANdbFile=D:\desktop\enable.dbc  MsgList=(none)  MsgName=AMK_ActualValue1  MsgIDType=Standard (11-bit identifier)  MsgIdentifier=643  MsgLength=8  Remote=off  ApplyMinMax=off  BusOutput=off  SignalInfo={'AMK_ActualVelocity','16','16','LE','signed','Standard','0','1','0','0','65535';'AMK_MagnetizingCurrent','48','16','LE','signed','Standard','0','1','0','0','65535';'AMK_TorqueCurrent','32','16','LE','signed','Standard','0','1','0','0','65535';'AMK_bDcOn1','12','1','LE','unsigned','Standard','0','1','0','0','1';'AMK_bDerating1','15','1','LE','unsigned','Standard','0','1','0','0','1';'AMK_bError1','9','1','LE','unsigned','Standard','0','1','0','0','1';'AMK_bInverterOn1','14','1','LE','unsigned','Standard','0','1','0','0','1';'AMK_bQuitDcOn1','11','1','LE','unsigned','Standard','0','1','0','0','1';'AMK_bQuitInverterOn1','13','1','LE','unsigned','Standard','0','1','0','0','1';'AMK_bReserve1','0','8','LE','unsigned','Standard','0','1','0','0','255';'AMK_bSystemReady1','8','1','LE','unsigned','Standard','0','1','0','0','1';'AMK_bWarn1','10','1','LE','unsigned','Standard','0','1','0','0','1'}
      settings: SourceProductBaseCode=ME,XP,VN  DataFormat=CANdb specified signals
  CAN Unpack : canmsglib/CAN Unpack  CANdbFile=C:\Users\86155\Desktop\HRT2024\qkx\can\enable.dbc  MsgList=AMK_ActualValue2  MsgName=AMK_ActualValue2  MsgIDType=Standard (11-bit identifier)  MsgIdentifier=645  MsgLength=8  SignalInfo={'AMK_ErrorInfo','32','16','LE','unsigned','Standard','0','1','0','0','65535';'AMK_TempIGBT','48','16','LE','signed','Standard','0','1','0','-32768','32767';'AMK_TempInverter','16','16','LE','signed','Standard','0','1','0','-32768','32767';'AMK_TempMotor','0','16','LE','signed','Standard','0','1','0','-32768','32767'}  IDPort=off  TimestampPort=off  ErrorPort=off  RemotePort=off  LengthPort=off  StatusPort=off  ApplyMinMax=off
      settings: SourceProductBaseCode=ME,XP,VN  DataFormat=CANdb specified signals
  CANPackMessage : ec5744lib/RapidECU_U4B/04CANCommunication/CANPackMessage  Commented=on  datalength=8  sampletime=-1
      settings: SourceProductName=ECUCoder for MPC5744
  CANUnPackMessage : ec5744lib/RapidECU_U4B/04CANCommunication/CANUnPackMessage  datalength=8  canmessagetype=Standard(11-bit ID)  sampletime=-1
      settings: SourceProductName=ECUCoder for MPC5744
  wires:
  msg/1 -> CANUnPackMessage/2
  CANUnPackMessage/1 -> CAN Unpack/1
  ID/1 -> CANUnPackMessage/1
  CANPackMessage/1 -> ?
  CAN Pack/1 -> CANPackMessage/1

== system control/Subsystem/Rx/284 286右前/Subsystem2/Subsystem ==
  ID : Inport
  msg : Inport  Port=2
  Enable : EnablePort
  CAN Pack : canmsglib/CAN Pack  Commented=on  CANdbFile=D:\desktop\enable.dbc  MsgList=(none)  MsgName=AMK_ActualValue1  MsgIDType=Standard (11-bit identifier)  MsgIdentifier=643  MsgLength=8  Remote=off  ApplyMinMax=off  BusOutput=off  SignalInfo={'AMK_ActualVelocity','16','16','LE','signed','Standard','0','1','0','0','65535';'AMK_MagnetizingCurrent','48','16','LE','signed','Standard','0','1','0','0','65535';'AMK_TorqueCurrent','32','16','LE','signed','Standard','0','1','0','0','65535';'AMK_bDcOn1','12','1','LE','unsigned','Standard','0','1','0','0','1';'AMK_bDerating1','15','1','LE','unsigned','Standard','0','1','0','0','1';'AMK_bError1','9','1','LE','unsigned','Standard','0','1','0','0','1';'AMK_bInverterOn1','14','1','LE','unsigned','Standard','0','1','0','0','1';'AMK_bQuitDcOn1','11','1','LE','unsigned','Standard','0','1','0','0','1';'AMK_bQuitInverterOn1','13','1','LE','unsigned','Standard','0','1','0','0','1';'AMK_bReserve1','0','8','LE','unsigned','Standard','0','1','0','0','255';'AMK_bSystemReady1','8','1','LE','unsigned','Standard','0','1','0','0','1';'AMK_bWarn1','10','1','LE','unsigned','Standard','0','1','0','0','1'}
      settings: SourceProductBaseCode=ME,XP,VN  DataFormat=CANdb specified signals
  CAN Unpack : canmsglib/CAN Unpack  CANdbFile=C:\Users\86155\Desktop\HRT2024\qkx\can\enable.dbc  MsgList=AMK_ActualValue1  MsgName=AMK_ActualValue1  MsgIDType=Standard (11-bit identifier)  MsgIdentifier=643  MsgLength=8  SignalInfo={'AMK_ActualVelocity','16','16','LE','signed','Standard','0','1','0','-32768','32767';'AMK_MagnetizingCurrent','48','16','LE','signed','Standard','0','1','0','-32768','32767';'AMK_TorqueCurrent','32','16','LE','signed','Standard','0','1','0','-32768','32767';'AMK_bDcOn1','12','1','LE','unsigned','Standard','0','1','0','0','1';'AMK_bDerating1','15','1','LE','unsigned','Standard','0','1','0','0','1';'AMK_bError1','9','1','LE','unsigned','Standard','0','1','0','0','1';'AMK_bInverterOn1','14','1','LE','unsigned','Standard','0','1','0','0','1';'AMK_bQuitDcOn1','11','1','LE','unsigned','Standard','0','1','0','0','1';'AMK_bQuitInverterOn1','13','1','LE','unsigned','Standard','0','1','0','0','1';'AMK_bReserve1','0','8','LE','unsigned','Standard','0','1','0','0','255';'AMK_bSystemReady1','8','1','LE','unsigned','Standard','0','1','0','0','1';'AMK_bWarn1','10','1','LE','unsigned','Standard','0','1','0','0','1'}  IDPort=off  TimestampPort=off  ErrorPort=off  RemotePort=off  LengthPort=off  StatusPort=off  ApplyMinMax=off
      settings: SourceProductBaseCode=ME,XP,VN  DataFormat=CANdb specified signals
  CANPackMessage : ec5744lib/RapidECU_U4B/04CANCommunication/CANPackMessage  Commented=on  datalength=8  sampletime=-1
      settings: SourceProductName=ECUCoder for MPC5744
  CANUnPackMessage : ec5744lib/RapidECU_U4B/04CANCommunication/CANUnPackMessage  datalength=8  canmessagetype=Standard(11-bit ID)  sampletime=-1
      settings: SourceProductName=ECUCoder for MPC5744
  Data Store Write : DataStoreWrite  DataStoreName=dianji_velcoity_youqian
  Data Store Write1 : DataStoreWrite  DataStoreName=er_v_rf
  Data Store Write2 : DataStoreWrite  DataStoreName=er_T_rf
  MATLAB Function : MATLAB Function  TreatAsAtomicUnit=on
  wires:
  msg/1 -> CANUnPackMessage/2
  CANUnPackMessage/1 -> CAN Unpack/1
  ID/1 -> CANUnPackMessage/1
  CANPackMessage/1 -> ?
  CAN Pack/1 -> CANPackMessage/1
  CAN Unpack/1 -> Data Store Write1/1, MATLAB Function/1(u)
  MATLAB Function/1(y) -> Data Store Write/1
  CAN Unpack/3 -> Data Store Write2/1

== system control/Subsystem/Rx/287 289右后/Subsystem1/Subsystem ==
  ID : Inport
  msg : Inport  Port=2
  Enable : EnablePort
  CAN Pack : canmsglib/CAN Pack  Commented=on  CANdbFile=D:\desktop\enable.dbc  MsgList=(none)  MsgName=AMK_ActualValue1  MsgIDType=Standard (11-bit identifier)  MsgIdentifier=643  MsgLength=8  Remote=off  ApplyMinMax=off  BusOutput=off  SignalInfo={'AMK_ActualVelocity','16','16','LE','signed','Standard','0','1','0','0','65535';'AMK_MagnetizingCurrent','48','16','LE','signed','Standard','0','1','0','0','65535';'AMK_TorqueCurrent','32','16','LE','signed','Standard','0','1','0','0','65535';'AMK_bDcOn1','12','1','LE','unsigned','Standard','0','1','0','0','1';'AMK_bDerating1','15','1','LE','unsigned','Standard','0','1','0','0','1';'AMK_bError1','9','1','LE','unsigned','Standard','0','1','0','0','1';'AMK_bInverterOn1','14','1','LE','unsigned','Standard','0','1','0','0','1';'AMK_bQuitDcOn1','11','1','LE','unsigned','Standard','0','1','0','0','1';'AMK_bQuitInverterOn1','13','1','LE','unsigned','Standard','0','1','0','0','1';'AMK_bReserve1','0','8','LE','unsigned','Standard','0','1','0','0','255';'AMK_bSystemReady1','8','1','LE','unsigned','Standard','0','1','0','0','1';'AMK_bWarn1','10','1','LE','unsigned','Standard','0','1','0','0','1'}
      settings: SourceProductBaseCode=ME,XP,VN  DataFormat=CANdb specified signals
  CAN Unpack : canmsglib/CAN Unpack  CANdbFile=C:\Users\86155\Desktop\HRT2024\qkx\can\enable.dbc  MsgList=AMK_ActualValue2  MsgName=AMK_ActualValue2  MsgIDType=Standard (11-bit identifier)  MsgIdentifier=645  MsgLength=8  SignalInfo={'AMK_ErrorInfo','32','16','LE','unsigned','Standard','0','1','0','0','65535';'AMK_TempIGBT','48','16','LE','signed','Standard','0','1','0','-32768','32767';'AMK_TempInverter','16','16','LE','signed','Standard','0','1','0','-32768','32767';'AMK_TempMotor','0','16','LE','signed','Standard','0','1','0','-32768','32767'}  IDPort=off  TimestampPort=off  ErrorPort=off  RemotePort=off  LengthPort=off  StatusPort=off  ApplyMinMax=off
      settings: SourceProductBaseCode=ME,XP,VN  DataFormat=CANdb specified signals
  CANPackMessage : ec5744lib/RapidECU_U4B/04CANCommunication/CANPackMessage  Commented=on  datalength=8  sampletime=-1
      settings: SourceProductName=ECUCoder for MPC5744
  CANUnPackMessage : ec5744lib/RapidECU_U4B/04CANCommunication/CANUnPackMessage  datalength=8  canmessagetype=Standard(11-bit ID)  sampletime=-1
      settings: SourceProductName=ECUCoder for MPC5744
  wires:
  msg/1 -> CANUnPackMessage/2
  CANUnPackMessage/1 -> CAN Unpack/1
  ID/1 -> CANUnPackMessage/1
  CANPackMessage/1 -> ?
  CAN Pack/1 -> CANPackMessage/1
